simulink model "Basic_3DoF_Delta_2021a"  (R2021a)
settings: Solver=ode4  StartTime=0.0  StopTime=time(end)  FixedStep=0.001  RelTol=1e-6
model workspace: external: MATLAB File robot_6kg_v4_EXa5_DataFile.m (data not in the file)
values from neighbouring files (symbols this model uses):
  IAB = (Im + IA + IB)    [Basic_3DoF_Delta_Dynamic_Param.m]    (also in RL5_6kg_Dynamic_Param.m)
  IABe = (Im + IA + IBe)    [Basic_3DoF_Delta_Dynamic_Param.m]
  lB = l1*(rho1*m1 + me)    [Basic_3DoF_Delta_Dynamic_Param.m]    (also in RL5_6kg_Dynamic_Param.m)
  lBe = l1*(m1/2 + me)    [Basic_3DoF_Delta_Dynamic_Param.m]
  mD = m3 + 3*m2 + 3*me    [Basic_3DoF_Delta_Dynamic_Param.m]    (also in RL5_6kg_Dynamic_Param.m = m3 + 3*m2 + 3*me + mls_a4_spi + mls_a5_spi + mls_a5_worm)
  rho2 = Sro2    [Basic_3DoF_Delta_Dynamic_Param.m]    (also in RL5_6kg_Dynamic_Param.m)
undefined symbols (not defined in the file or in its folder): Inertias, X, Y, Z
libraries: sm_lib x119, nesl_utility x19, eeGeneralControl x3, simulink x3
(part 1 of 4)
settings Model: Creator=SUSTRVOJ  LastModifiedBy=baran.alikoc
settings SolverCC: AlgebraicLoopSolver=TrustRegion
settings DataIOCC: SaveOutput=off  SignalLogging=off  DSMLogging=off  SaveTime=off  ReturnWorkspaceOutputs=off
settings DebuggingCC: SFMachineParentedDataDiag=warning
settings DiagnosticsConfigSet: SimMechanicsJointTargetOverSpecification=warning
settings ExplorerConfigSet: InternalSimMechanicsExplorerSettings="<ExplorerConfiguration><canonicalview>default</canonicalview><AnimationSetting><BasePlaybackSpeed>1.0</BasePlaybackSpeed><PlaybackSpeedFactor>1.0</PlaybackSpeedFactor></AnimationSetting><TilePanel><TileInfo><Tiles Columns=\"1\" Count=\"1\" Rows=\"1\"><Column Weight=\"1\"/><Row Weight=\"1\"/><Tile Height=\"1\" Width=\"1\" X=\"0\" Y=\"0\"/></Tiles></TileInfo><SceneInfo><SceneViewer><BGColor><R>0.60000002384185791</R><G>0.60000002384185791</G><B>0.60000002384185791</B></BGColor><Camera><DoPerspective>off</DoPerspective><Position><X>0.135215272225856747</X><Y>-1.20095496527992429</Y><Z>-0.491222676043407747</Z></Position><Center><X>0.135215272225856747</X><Y>5.5511151231257827e-17</Y><Z>-0.491222676043407747</Z></Center><Up><X>0</X><Y>-0</Y><Z>1</Z></Up><ViewLimDist>1</ViewLimDist><YLim>0.916798880077600797</YLim><XLim>1.0012025864974432</XLim></Camera></SceneViewer></SceneInfo></TilePanel><MechEditorPanel><Cameras/><GfxPanelCameraMap/><VideoCreator><PlaybackSpeedRatio>1.0</PlaybackSpeedRatio><FrameRate>30</FrameRate><VideoFormat>Motion JPEG AVI</VideoFormat><FrameSize>auto</FrameSize></VideoCreator></MechEditorPanel></ExplorerConfiguration>"

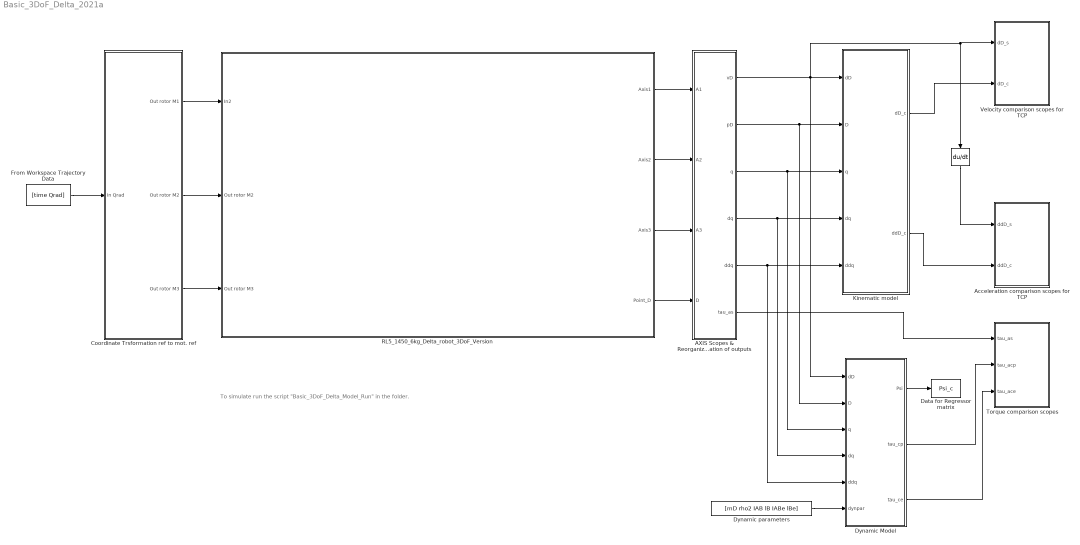
== system Basic_3DoF_Delta_2021a ==
  note: To simulate run the script "Basic_3DoF_Delta_Model_Run" in the folder.
  "   " : Derivative
  AXIS Scopes & Reorganization of outputs : Subsystem
  Acceleration comparison scopes for TCP : Subsystem
  Coordinate Trsformation ref to mot. ref : Subsystem
  Data for Regressor matrix : ToWorkspace  VariableName=Psi_c  SaveFormat=Structure With Time  SampleTime=-1
  Dynamic Model : MATLAB Function  TreatAsAtomicUnit=on
  Dynamic parameters : Constant  Value=[mD rho2 IAB lB IABe lBe]
  From Workspace Trajectory Data : FromWorkspace  VariableName=[time Qrad]  SampleTime=1e-3
  Kinematic model : MATLAB Function  TreatAsAtomicUnit=on
  RL5_1450_6kg_Delta_robot_3DoF_Version : Subsystem
  Torque comparison scopes : Subsystem
  Velocity comparison scopes for TCP : Subsystem
  wires:
  From Workspace Trajectory Data/1 -> Coordinate Trsformation ref to mot. ref/1(In Qrad)
  Coordinate Trsformation ref to mot. ref/1(Out rotor M1) -> RL5_1450_6kg_Delta_robot_3DoF_Version/1(In2)
  Coordinate Trsformation ref to mot. ref/2(Out rotor M2) -> RL5_1450_6kg_Delta_robot_3DoF_Version/2(Out rotor M2)
  Coordinate Trsformation ref to mot. ref/3(Out rotor M3) -> RL5_1450_6kg_Delta_robot_3DoF_Version/3(Out rotor M3)
  RL5_1450_6kg_Delta_robot_3DoF_Version/4(Point_D) -> AXIS Scopes & Reorganization of outputs/4(D)
  RL5_1450_6kg_Delta_robot_3DoF_Version/3(Axis3) -> AXIS Scopes & Reorganization of outputs/3(A3)
  RL5_1450_6kg_Delta_robot_3DoF_Version/2(Axis2) -> AXIS Scopes & Reorganization of outputs/2(A2)
  RL5_1450_6kg_Delta_robot_3DoF_Version/1(Axis1) -> AXIS Scopes & Reorganization of outputs/1(A1)
  Dynamic Model/2(tau_cp) -> Torque comparison scopes/2(tau_acp)
  Dynamic parameters/1 -> Dynamic Model/6(dynpar)
  Dynamic Model/1(Psi) -> Data for Regressor matrix/1
  Kinematic model/2(ddD_c) -> Acceleration comparison scopes for TCP/2(ddD_c)
  "   "/1 -> Acceleration comparison scopes for TCP/1(ddD_s)
  AXIS Scopes & Reorganization of outputs/2(pD) -> Dynamic Model/2(D), Kinematic model/2(D)
  AXIS Scopes & Reorganization of outputs/3(q) -> Dynamic Model/3(q), Kinematic model/3(q)
  AXIS Scopes & Reorganization of outputs/4(dq) -> Dynamic Model/4(dq), Kinematic model/4(dq)
  AXIS Scopes & Reorganization of outputs/5(ddq) -> Dynamic Model/5(ddq), Kinematic model/5(ddq)
  AXIS Scopes & Reorganization of outputs/6(tau_as) -> Torque comparison scopes/1(tau_as)
  AXIS Scopes & Reorganization of outputs/1(vD) -> Dynamic Model/1(dD), Kinematic model/1(dD), "   "/1, Velocity comparison scopes for TCP/1(dD_s)
  Kinematic model/1(dD_c) -> Velocity comparison scopes for TCP/2(dD_c)
  Dynamic Model/3(tau_ce) -> Torque comparison scopes/3(tau_ace)

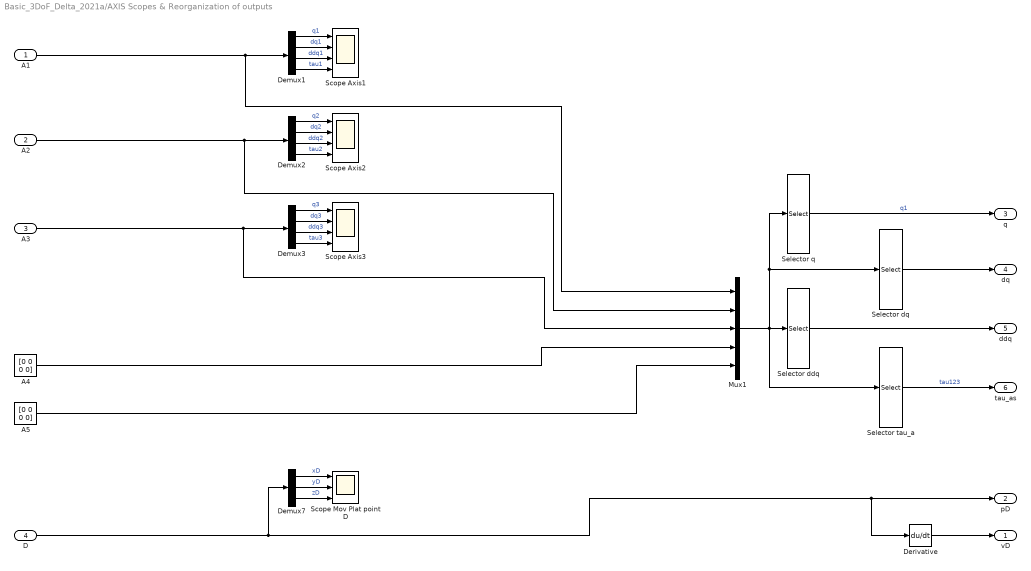
== system Basic_3DoF_Delta_2021a/AXIS Scopes & Reorganization of outputs ==
  A1 : Inport
  A2 : Inport  Port=2
  A3 : Inport  Port=3
  D : Inport  Port=4
  A4 : Constant  Value=[0 0 0 0]
  A5 : Constant  Value=[0 0 0 0]
  Demux1 : Demux
  Demux2 : Demux
  Demux3 : Demux
  Demux7 : Demux  Outputs=3
  Derivative : Derivative
  Mux1 : Mux  Inputs=5
  Scope Axis1 : Scope  NumInputPorts=4
  Scope Axis2 : Scope  NumInputPorts=4
  Scope Axis3 : Scope  NumInputPorts=4
  Scope Mov Plat point D : Scope  NumInputPorts=3
  Selector ddq : Selector  InputPortWidth=20  IndexOptions=Index vector (dialog)  Indices=[3 7 11 15 19]  OutputSizes=1
  Selector dq : Selector  InputPortWidth=20  IndexOptions=Index vector (dialog)  Indices=[2 6 10 14 18]  OutputSizes=1
  Selector q : Selector  InputPortWidth=20  IndexOptions=Index vector (dialog)  Indices=[1 5 9 13 17]  OutputSizes=1
  Selector tau_a : Selector  InputPortWidth=20  IndexOptions=Index vector (dialog)  Indices=[4 8 12]  OutputSizes=1
  vD : Outport
  pD : Outport  Port=2
  q : Outport  Port=3
  dq : Outport  Port=4
  ddq : Outport  Port=5
  tau_as : Outport  Port=6
  wires:
  A4/1 -> Mux1/4
  A1/1 -> Mux1/1, Demux1/1
  A5/1 -> Mux1/5
  D/1 -> Demux7/1, Derivative/1, pD/1
  Demux3/2 -> Scope Axis3/2  "dq3"
  Demux3/3 -> Scope Axis3/3  "ddq3"
  Demux7/1 -> Scope Mov Plat point D/1  "xD"
  Demux7/3 -> Scope Mov Plat point D/3  "zD"
  Demux3/4 -> Scope Axis3/4  "tau3"
  Demux2/1 -> Scope Axis2/1  "q2"
  Demux7/2 -> Scope Mov Plat point D/2  "yD"
  Demux3/1 -> Scope Axis3/1  "q3"
  A3/1 -> Mux1/3, Demux3/1
  Demux2/4 -> Scope Axis2/4  "tau2"
  Demux1/4 -> Scope Axis1/4  "tau1"
  A2/1 -> Mux1/2, Demux2/1
  Demux2/2 -> Scope Axis2/2  "dq2"
  Demux2/3 -> Scope Axis2/3  "ddq2"
  Demux1/1 -> Scope Axis1/1  "q1"
  Demux1/3 -> Scope Axis1/3  "ddq1"
  Demux1/2 -> Scope Axis1/2  "dq1"
  Selector ddq/1 -> ddq/1
  Selector q/1 -> q/1  "q1"
  Mux1/1 -> Selector ddq/1, Selector dq/1, Selector q/1, Selector tau_a/1
  Selector dq/1 -> dq/1
  Selector tau_a/1 -> tau_as/1  "tau123"
  Derivative/1 -> vD/1

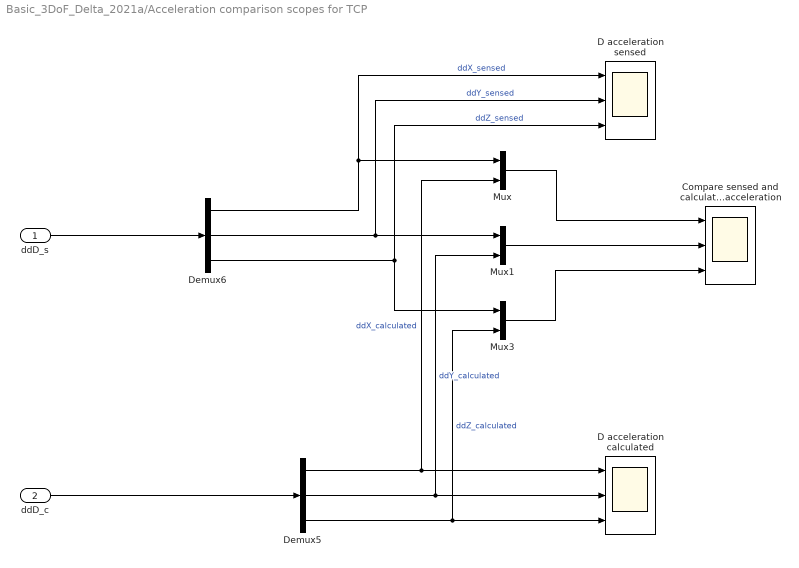
== system Basic_3DoF_Delta_2021a/Acceleration comparison scopes for TCP ==
  ddD_s : Inport
  ddD_c : Inport  Port=2
  Compare sensed and calculated D acceleration : Scope  NumInputPorts=3
  D acceleration calculated : Scope  NumInputPorts=3
  D acceleration sensed : Scope  NumInputPorts=3
  Demux5 : Demux  Outputs=3
  Demux6 : Demux  Outputs=3
  Mux : Mux  Inputs=2
  Mux1 : Mux  Inputs=2
  Mux3 : Mux  Inputs=2
  wires:
  Demux6/3 -> D acceleration sensed/3, Mux3/1  "ddZ_sensed"
  Demux5/3 -> Mux3/2, D acceleration calculated/3  "ddZ_calculated"
  Demux5/2 -> D acceleration calculated/2, Mux1/2  "ddY_calculated"
  Demux6/2 -> D acceleration sensed/2, Mux1/1  "ddY_sensed"
  Demux6/1 -> D acceleration sensed/1, Mux/1  "ddX_sensed"
  ddD_s/1 -> Demux6/1
  Demux5/1 -> D acceleration calculated/1, Mux/2  "ddX_calculated"
  Mux1/1 -> Compare sensed and calculated D acceleration/2
  Mux3/1 -> Compare sensed and calculated D acceleration/3
  Mux/1 -> Compare sensed and calculated D acceleration/1
  ddD_c/1 -> Demux5/1

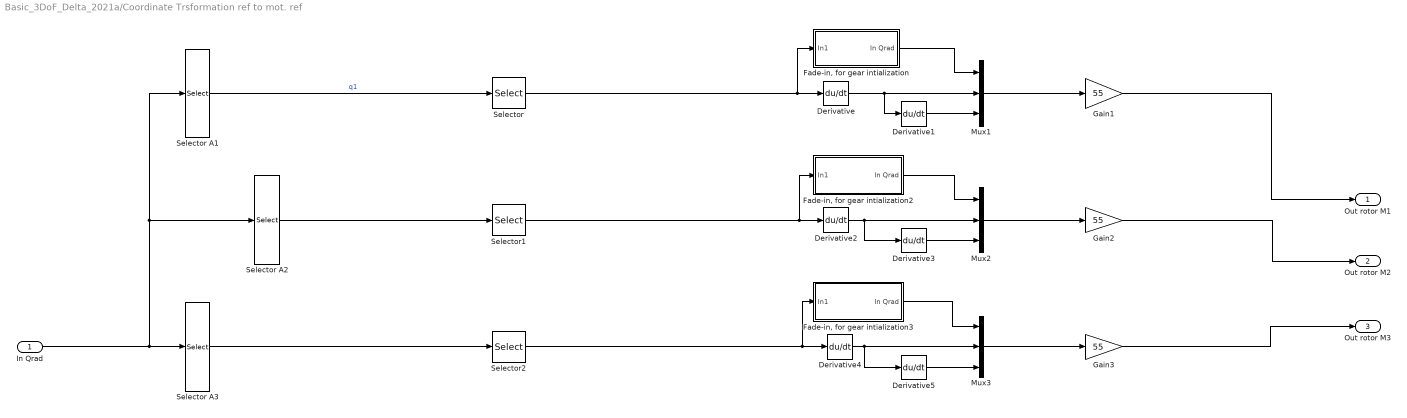
== system Basic_3DoF_Delta_2021a/Coordinate Trsformation ref to mot. ref ==
  In Qrad : Inport
  Derivative{,1..5} (6 alike) : Derivative
  "Fade-in, for gear intialization" : Subsystem
  "Fade-in, for gear intialization2" : Subsystem
  "Fade-in, for gear intialization3" : Subsystem
  Gain1 : Gain  Gain=55
  Gain2 : Gain  Gain=55
  Gain3 : Gain  Gain=55
  Mux1 : Mux  Inputs=3
  Mux2 : Mux  Inputs=3
  Mux3 : Mux  Inputs=3
  Selector : Selector  InputPortWidth=3  IndexOptions=Index vector (dialog)  Indices=[1]  OutputSizes=1
  Selector A1 : Selector  InputPortWidth=15  IndexOptions=Index vector (dialog)  Indices=[1 6 11]  OutputSizes=1
  Selector A2 : Selector  InputPortWidth=15  IndexOptions=Index vector (dialog)  Indices=[2 7 12]  OutputSizes=1
  Selector A3 : Selector  InputPortWidth=15  IndexOptions=Index vector (dialog)  Indices=[3 8 13]  OutputSizes=1
  Selector1 : Selector  InputPortWidth=3  IndexOptions=Index vector (dialog)  Indices=[1]  OutputSizes=1
  Selector2 : Selector  InputPortWidth=3  IndexOptions=Index vector (dialog)  Indices=[1]  OutputSizes=1
  Out rotor M1 : Outport
  Out rotor M2 : Outport  Port=2
  Out rotor M3 : Outport  Port=3
  wires:
  In Qrad/1 -> Selector A1/1, Selector A2/1, Selector A3/1
  Gain1/1 -> Out rotor M1/1
  Gain2/1 -> Out rotor M2/1
  Gain3/1 -> Out rotor M3/1
  Derivative1/1 -> Mux1/3
  Derivative/1 -> Mux1/2, Derivative1/1
  Selector A1/1 -> Selector/1  "q1"
  Mux1/1 -> Gain1/1
  Mux2/1 -> Gain2/1
  Mux3/1 -> Gain3/1
  Derivative3/1 -> Mux2/3
  Derivative2/1 -> Mux2/2, Derivative3/1
  Derivative5/1 -> Mux3/3
  Derivative4/1 -> Mux3/2, Derivative5/1
  Selector2/1 -> "Fade-in, for gear intialization3"/1(In1), Derivative4/1
  Selector1/1 -> "Fade-in, for gear intialization2"/1(In1), Derivative2/1
  Selector/1 -> "Fade-in, for gear intialization"/1(In1), Derivative/1
  Selector A3/1 -> Selector2/1
  "Fade-in, for gear intialization"/1(In Qrad) -> Mux1/1
  Selector A2/1 -> Selector1/1
  "Fade-in, for gear intialization2"/1(In Qrad) -> Mux2/1
  "Fade-in, for gear intialization3"/1(In Qrad) -> Mux3/1
